simulink model "LAB_2_GROUP_1_2_2"  (R2019a)
settings: Solver=VariableStepAuto  StartTime=0.0  StopTime=10.0  RelTol=1e-3
libraries: simulink x1
settings Model: Creator=fiado  LastModifiedBy=fiado

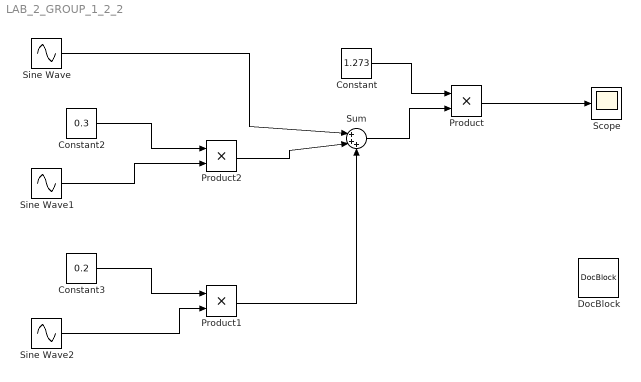
== system LAB_2_GROUP_1_2_2 ==
  Constant : Constant  Value=1.273
  Constant2 : Constant  Value=0.3
  Constant3 : Constant  Value=0.2
  DocBlock : simulink/Model-Wide Utilities/DocBlock  DocumentType=Text
      content=|
      | Simulation of  signal
      | x(t) = (4/pi)*[sin(t) + 1/3 * sin(3t) + 1/5 * sin(5t)]
      | Simulation Details:
      | - Simulation Time : 10 seconds
      |
      | Description:
      | This Simulink model demonstrates the signal x(t)
      |
      | Model Overview:
      | - The "Sine Wave" block generates the sine wave (sin(t))
      | - The "Sine Wave 1" block generates the sine wave (sin(3t))
      | - The "Sine Wave 2" block generates the sine wave (sin(5t))
      | - The "Product" block combines the constant block
      |  (0.3) with the sine wave (sin(3t))
      | - Another "Product" block combines the other constant block
      |  (0.2) with the sine wave (sin(5t))
      | - The results from the two product blocks are combined
      |   with the sine wave (sin(t))using the "Sum" block
      | - The result from the sum block is combined with the
      |   constant block (1.273) using a "Product" block
      | - The results are then displayed on a "Scope" block.
  Product : Product
  Product1 : Product
  Product2 : Product
  Scope : Scope
  Sine Wave : Sin  Frequency=0.159  SampleTime=0
  Sine Wave1 : Sin  Frequency=0.477  SampleTime=0
  Sine Wave2 : Sin  Frequency=0.795  SampleTime=0
  Sum : Sum  Inputs=|+++
  wires:
  Constant2/1 -> Product2/1
  Sine Wave1/1 -> Product2/2
  Constant3/1 -> Product1/1
  Sine Wave2/1 -> Product1/2
  Product2/1 -> Sum/2
  Product1/1 -> Sum/3
  Sine Wave/1 -> Sum/1
  Constant/1 -> Product/1
  Sum/1 -> Product/2
  Product/1 -> Scope/1
